simulink model "uavModelModified_2018a"  (R2018a)
settings: Solver=VariableStepAuto  StartTime=0.0  StopTime=25  RelTol=1e-3
undefined symbols (not defined in the file or in its folder): Motor
libraries: simulink x8
(part 2 of 2)

== matlab function uavModelModified_2018a/wind_simulator/wind_and_gust/MATLAB Function ==
  data: direction input; wind output; speed input; enabled input; t input
function wind = wind_generator(direction, speed, enabled, t)
%
% direction: 1 for tail wind, -1 for headwind
% speed: in m/s
%
wind = [0,0,0];

if enabled
    if direction ~= 1 && direction ~= -1
        error("direction should be 1 for tail wind or -1 for headwind");
    end
    if speed < 0 && speed > 5
        error("speed should be between 0 and 5");
    end
    wind(2) = direction * speed;
end

== matlab function uavModelModified_2018a/PID_Controller_PitchRollYawAltitude/MATLAB Function ==
  data: speed input; pitch output
function pitch  = speed2pitch(speed)

    pitch = (2.10471847e-03)*speed + (5.35884537e-05)*speed^2;
    pitch = pitch - pitch*.27;
    pitch = round(pitch*1000)/1000; %rounds to 3rd decimal

== matlab function uavModelModified_2018a/PID_Controller_PitchRollYawAltitude/MATLAB Function1 ==
  data: t input; cur_y_vel input; pitch output; cur_pitch input; pitch_ref input; cur_y_pos input; y_pos_ref input
function pitch = pitchController(t, cur_y_vel, cur_pitch,pitch_ref, cur_y_pos, y_pos_ref)

MAX_VEL = 6.0;
k_pitch = 1.0;
c_pitch = 1.0

if t < 5
    pitch = 0.0;
else
    % velocity checks
    if cur_y_vel < .6 * MAX_VEL
        k_pitch = .5;
    elseif cur_y_vel >= .6 * MAX_VEL && cur_y_vel < .7 * MAX_VEL
        k_pitch = .1;
    elseif cur_y_vel >= .7 * MAX_VEL && cur_y_vel < .8 * MAX_VEL
        k_pitch = .05;
    elseif cur_y_vel >= .8 * MAX_VEL && cur_y_vel < MAX_VEL
        k_pitch = 0.0;
    else
        pitch = -.0001;
        return;
    end
    
    % position checks
    if cur_y_pos < .6 * y_pos_ref
        c_pitch = .50;
    elseif cur_y_pos >= .6 * y_pos_ref && cur_y_pos < .7 * y_pos_ref
        c_pitch = .1;
    elseif cur_y_pos >= .7 * y_pos_ref && cur_y_pos < .8 * y_pos_ref
        c_pitch = .05;
    elseif cur_y_pos >= .8 * y_pos_ref && cur_y_pos < y_pos_ref
        pitch = 0.0;
        return;
    else
        pitch = -.0001;
        return;
    end
        
    pitch = k_pitch * pitch_ref * c_pitch;
end

== matlab function uavModelModified_2018a/MATLAB Function ==
  data: t input; pitch_out output; pitch_ref input
function pitch_out = pitchRef(t, pitch_ref)


    if t > 10 && t < 15
        pitch_out = pitch_ref;
    else
        pitch_out = 0.000;
    end

== matlab function uavModelModified_2018a/motors2/BLDC Motor3/Propeller model  ==
  data: torque output; rpm input; thrust output
function [torque,thrust] = fcn(rpm)
% angular_velocity in rpm

%coefficient of thrust, empirically derived
coef_t = 2*(10^-15)*rpm^3 - 4*(10^-11)*rpm^2 + 3*(10^-7)*rpm + .1013;
%thrust = coef_t * density of air * velocity^2 * propeller diameter (m) ^4
thrust = coef_t*1.225*(rpm/60)^2*.2^4;
% empirically derived
torque = 4*(10^-14)*rpm^3 +  8*(10^-12)*rpm^2 + 3*(10^-6)*rpm;
end
